simulink model "Model_01_work_2017_contr"  (R2017a)
settings: Solver=FixedStepAuto  StartTime=0.0  StopTime=96  FixedStep=0.01  RelTol=1e-3
settings Model: Creator=alexandr.lanin  LastModifiedBy=alexandr.lanin
settings DataIOCC: SaveFormat=StructureWithTime
settings OptimizationCC: DefaultUnderspecifiedDataType=single
settings ConfigComp: CovScope=ReferencedModels  CovIncludeTopModel=off

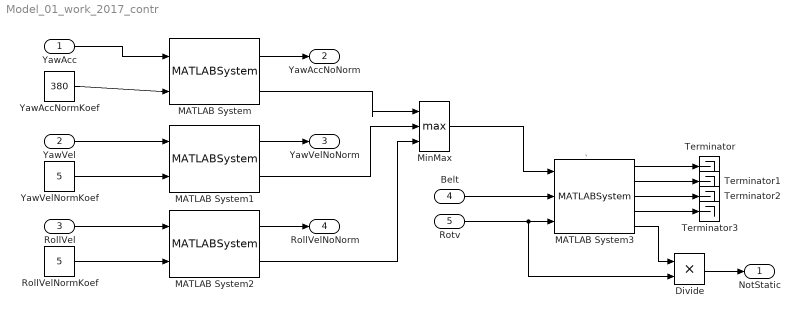
== system Model_01_work_2017_contr ==
  note: `
  YawAcc : Inport  OutDataTypeStr=double
  YawVel : Inport  Port=2  OutDataTypeStr=double
  RollVel : Inport  Port=3  OutDataTypeStr=double
  Belt : Inport  Port=4  OutDataTypeStr=double
  Rotv : Inport  Port=5  OutDataTypeStr=double
  Divide : Product  Inputs=**
  MATLAB System : MATLABSystem  System=WolchSimCode  kMul=100  SimulateUsing=Code generation
      mask Type: WolchSimCode
      mask Display:
      | disp('WolchSimCode');
      | port_label('input',1,'u');
      | port_label('input',2,'norm');
      | port_label('output',1,'Y');
      | port_label('output',2,'Ynorm');
  MATLAB System1 : MATLABSystem  System=WolchSimCode  kMul=100  SimulateUsing=Code generation
      mask Type: WolchSimCode
      mask Display:
      | disp('WolchSimCode');
      | port_label('input',1,'u');
      | port_label('input',2,'norm');
      | port_label('output',1,'Y');
      | port_label('output',2,'Ynorm');
  MATLAB System2 : MATLABSystem  System=WolchSimCode  kMul=100  SimulateUsing=Code generation
      mask Type: WolchSimCode
      mask Display:
      | disp('WolchSimCode');
      | port_label('input',1,'u');
      | port_label('input',2,'norm');
      | port_label('output',1,'Y');
      | port_label('output',2,'Ynorm');
  MATLAB System3 : MATLABSystem  System=ModulSigmoid  Rwheel=17*0.0254  Transfer=3  Kreset=0.6  sd=6  sdsn=0.25  betta=0.6  sm_bet=0.3  alfa=1.0  sm_alfa=0.3  kStd=4  alfaExp=0.75  SimulateUsing=Code generation
      mask Type: ModulSigmoid
      mask Display:
      | disp('ModulSigmoid');
      | port_label('input',1,'signal');
      | port_label('input',2,'vBelt');
      | port_label('input',3,'rotv');
      | port_label('output',1,'y');
      | port_label('output',2,'k');
      | port_label('output',3,'v');
      | port_label('output',4,'ye');
      | port_label('output',5,'yinver');
  MinMax : MinMax  Function=max  Inputs=3
  RollVelNormKoef : Constant  Value=5
  Terminator{,1..3} (4 alike) : Terminator
  YawAccNormKoef : Constant  Value=380
  YawVelNormKoef : Constant  Value=5
  NotStatic : Outport  OutDataTypeStr=double
  YawAccNoNorm : Outport  Port=2  OutDataTypeStr=double
  YawVelNoNorm : Outport  Port=3  OutDataTypeStr=double
  RollVelNoNorm : Outport  Port=4  OutDataTypeStr=double
  wires:
  YawAcc/1 -> MATLAB System/1
  MATLAB System/2 -> MinMax/1
  YawAccNormKoef/1 -> MATLAB System/2
  MATLAB System1/2 -> MinMax/2
  YawVelNormKoef/1 -> MATLAB System1/2
  YawVel/1 -> MATLAB System1/1
  MATLAB System2/2 -> MinMax/3
  RollVel/1 -> MATLAB System2/1
  RollVelNormKoef/1 -> MATLAB System2/2
  MinMax/1 -> MATLAB System3/1
  Belt/1 -> MATLAB System3/2
  Rotv/1 -> Divide/2, MATLAB System3/3
  MATLAB System3/5 -> Divide/1
  Divide/1 -> NotStatic/1
  MATLAB System/1 -> YawAccNoNorm/1
  MATLAB System1/1 -> YawVelNoNorm/1
  MATLAB System2/1 -> RollVelNoNorm/1
  MATLAB System3/1 -> Terminator/1
  MATLAB System3/2 -> Terminator1/1
  MATLAB System3/4 -> Terminator3/1
  MATLAB System3/3 -> Terminator2/1
